simulink model "DF001A_FltInj"  (R2013b)
settings: Solver=FixedStepDiscrete  StartTime=0.0  StopTime=1  FixedStep=.002  RelTol=1e-3
values from neighbouring files (symbols this model uses):
  ARCHGLBPRM_180OVERPI_ULS_F32 = DataDict.Constant    [DF001A_FltInj_DataDict.m]
  ARCHGLBPRM_2PI_ULS_F32 = DataDict.Constant    [DF001A_FltInj_DataDict.m]
  FLOATTOU0P16MULT_ULS_F32 = DataDict.Constant    [DF001A_FltInj_DataDict.m]
  TICNVN_MILLISECPERCNT_F32 = DataDict.Constant    [DF001A_FltInj_DataDict.m]
libraries: simulink x6, NxtrLim x2, NxtrAbslt x1, NxtrMath x1, FixdToFloat x1
(part 1 of 2)
settings Model: PauseTimes=0.198  Creator=qzwc4r  LastModifiedBy=lzz0tm
settings DataIOCC: LimitDataPoints=off  SaveFormat=Structure  ReturnWorkspaceOutputs=on
settings OptimizationCC: BlockReduction=off  InlineParams=on  ZeroExternalMemoryAtStartup=off  ZeroInternalMemoryAtStartup=off  OptimizeModelRefInitCode=on  LifeSpan=1
settings DebuggingCC: SignalInfNanChecking=error  SignalRangeChecking=warning  UnderspecifiedInitializationDetection=Simplified  SolverPrmCheckMsg=error  InheritedTsInSrcMsg=error  DiscreteInheritContinuousMsg=error  SingleTaskRateTransMsg=error  TasksWithSamePriorityMsg=error  SigSpecEnsureSampleTimeMsg=error  CheckMatrixSingularityMsg=error  IntegerOverflowMsg=error  ParameterUnderflowMsg=error  ParameterPrecisionLossMsg=error  ParameterTunabilityLossMsg=error  FixptConstUnderflowMsg=warning  FixptConstOverflowMsg=warning  VectorMatrixConversionMsg=error  SignalLabelMismatchMsg=error  UnconnectedInputMsg=error  UnconnectedOutputMsg=error  UnconnectedLineMsg=error  SFcnCompatibilityMsg=error  UniqueDataStoreMsg=warning  BusObjectLabelMismatch=error  RootOutportRequireBusObject=error  AssertControl=DisableAll  ModelReferenceIOMsg=error  ModelReferenceVersionMismatchMessage=warning  ModelReferenceIOMismatchMessage=error  ModelReferenceCSMismatchMessage=warning  ModelReferenceDataLoggingMessage=error  StateNameClashWarn=warning  StrictBusMsg=ErrorOnBusTreatedAsVector  NonBusSignalsTreatedAsBus=error  SFUnexpectedBacktrackingDiag=error  SFInvalidInputDataAccessInChartInitDiag=error  SFNoUnconditionalDefaultTransitionDiag=error  SFTransitionOutsideNaturalParentDiag=error  SFUnconditionalTransitionShadowingDiag=error  SFUndirectedBroadcastEventsDiag=error
settings ModelReferenceCC: ModelReferenceNumInstancesAllowed=Single
settings RTWCC: SystemTargetFile=autosar.tlc  GenCodeOnly=on  TemplateMakefile=ert_default_tmf  Description=AUTOSAR  GenerateReport=on  ProcessScript=autosar_make_rtw_hook  LaunchReport=on
settings CodeAppCC: GenerateComments=off  IgnoreCustomStorageClasses=off  CustomSymbolStrType=$N$R$M  CustomSymbolStrBlkIO=$N$M  SimulinkBlockComments=off
settings STFCustomTargetCC: ParMdlRefBuildCompliant=on  CompOptLevelCompliant=on  IncludeMdlTerminateFcn=off  CombineOutputUpdateFcns=on  SuppressErrorStatus=on  ERTFirstTimeCompliant=on  ERTCustomFileBanners=on  SupportNonFinite=off  SupportComplex=off  SupportContinuousTime=off  SupportNonInlinedSFcns=off  MATLABClassNameForMDSCustomization=Simulink.SoftwareTarget.ERTCustomization  AutosarCompliant=on  GRTInterface=off  SystemTargetFile=autosar.tlc
settings ERTTargetCC: CodeReplacementLibrary=ANSI_C  ConcurrentExecutionCompliant=off  IncludeMdlTerminateFcn=off  SuppressErrorStatus=on  SupportNonFinite=off  SupportComplex=off  ModelStepFunctionPrototypeControlCompliant=off  CPPClassGenCompliant=off  AutosarCompliant=on  InlinedParameterPlacement=NonHierarchical  ERTCustomFileTemplate=example_file_process.tlc  EnableUserReplacementTypes=on

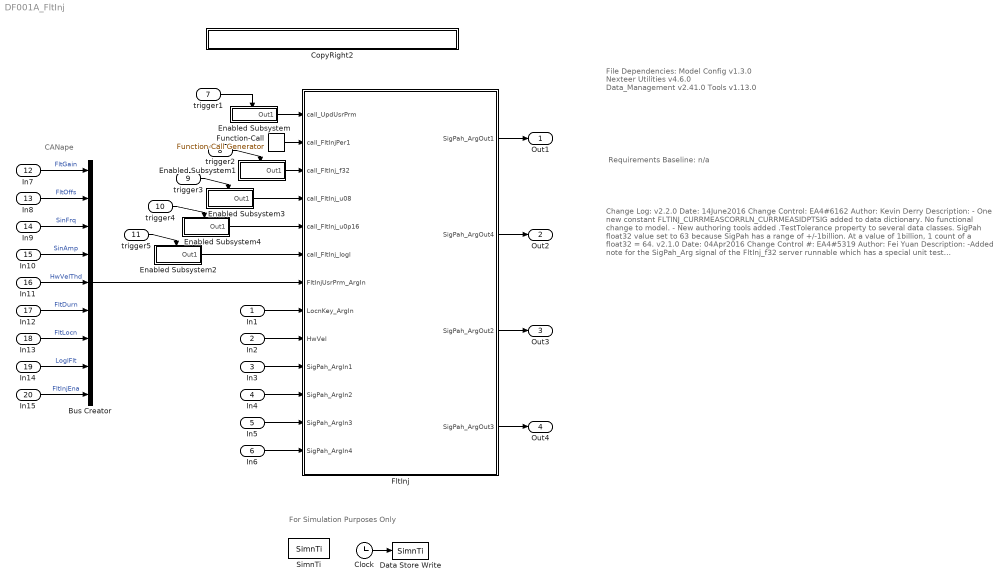
== system DF001A_FltInj ==
  note: CANape
  note: File Dependencies:
      |
      | Model Config v1.3.0
      | Nexteer Utilities v4.6.0
      | Data_Management v2.41.0
      | Tools v1.13.0
  note: Requirements Baseline: n/a
  note: Change Log:
      |
      | v2.2.0
      | Date: 14June2016
      | Change Control:  EA4#6162
      | Author:  Kevin Derry
      | Description:
      | - One new constant FLTINJ_CURRMEASCORRLN_CURRMEASIDPTSIG
      |   added to data dictionary.  No functional change to model.
      | - New authoring tools added .TestTolerance property to several data classes.
      |   SigPah float32 value set to 63 because SigPah has a range of +/-1billion.
      |   At a value of 1billion, 1 count of a float32 = 64.
      |
      | v2.1.0
      | Date: 04Apr2016
      | Change Control #: EA4#5319
      | Author: Fei Yuan
      | Description:
      | -Added note for the SigPah_Arg signal of the FltInj_f32 server runnable
      |  which has a special unit test consideration.
      | - Updated the range for the SigPah_Arg signal of the FltInj_u08 server
      |  runnable to 0-255.
      | - Removed the check for (FltInjUsrPrm.FltInjEna == TRUE) in the
      |   "else if" path.
      | - Added "Cnt" as the DocUnits of FltInjUsrPrm.
      |
      | v2.0.0
      | Change Control #:  EA4#3116
      | Author:  Kevin Derry
      | - New constant FLTINJ_TQOSCN_PREFINALCMD
      | - All constants .DocUnits changed from 'Uls' to 'Cnt' (should
      |   cause no effect on system)
      | - No functional changes to model.
      |
      | v1.1.0
      | Date: 26Aug2015
      | Change Control #: EA4#951
      | Author: Kevin Derry
      | Description:
      | - All InOut server arguments renamed to 'SigPah'.
      | - All PIM names now start with 'FltInj' because code is
      |     really using EA3-style module level variables.
      | - FLOATTOU0P16MULT_ULS_F32 was 65535, now 65536.
      | - Removed all requirements links.
      |
      | v1.0.0
      | Date: 21Aug2015
      | Change Control #: EA4#951
      | Author: Kevin Derry
      | Description:
      | - Initial Release
  note: For Simulation Purposes Only
  In1 : Inport
  In2 : Inport  Port=2
  In3 : Inport  Port=3
  In4 : Inport  Port=4
  In5 : Inport  Port=5
  In6 : Inport  Port=6
  trigger1 : Inport  Port=7
  trigger2 : Inport  Port=8
  trigger3 : Inport  Port=9
  trigger4 : Inport  Port=10
  trigger5 : Inport  Port=11
  In7 : Inport  Port=12
  In8 : Inport  Port=13
  In9 : Inport  Port=14
  In10 : Inport  Port=15
  In11 : Inport  Port=16
  In12 : Inport  Port=17
  In13 : Inport  Port=18
  In14 : Inport  Port=19
  In15 : Inport  Port=20
  Bus Creator : BusCreator  Inputs=9  OutDataTypeStr=Bus: FltInjUsrPrmRec1  NonVirtualBus=on
  Clock : Clock
  CopyRight2 : Subsystem  Description=|  mask(Copyright Information){none=on}
      | Copyright info block.                                               
      |                                                                     
      | Place copyright information at the top of every subsystem in design.
      mask prompts: none "No parameters"
      mask help: Place copyright information at the top of every subsystem in design.
      mask Display:
      | NxtrConf = 'Nexteer Confidential';
      | 
      | sys = bdroot; %handle for the current model ("system")
      | first = get_param(sys,'Created');
      | if(isempty(first))
      |     first = datestr(now,'yyyy');
      | else
      |     first = first(end-3:end);  %year is last four digits
      | end
      | 
      | last = get_param(sys,'LastModifiedDate');
      | if isempty(last)
      |     last = datestr(now,'yyyy');
      | else
      |     last = last(end-3:end);
      | end
      | 
      | if strcmp(first,last)
      |     fprintf('%s -- Copyright %s Nexteer',NxtrConf,first)
      | else
      |     fprintf('%s -- %s%s- %s Nexteer',NxtrConf,char(169),first,last)
      | end
  Data Store Write : DataStoreWrite  DataStoreName=SimnTi
  Enabled Subsystem : Subsystem  TreatAsAtomicUnit=on
  Enabled Subsystem1 : Subsystem  TreatAsAtomicUnit=on
  Enabled Subsystem2 : Subsystem  TreatAsAtomicUnit=on
  Enabled Subsystem3 : Subsystem  TreatAsAtomicUnit=on
  Enabled Subsystem4 : Subsystem  TreatAsAtomicUnit=on
  FltInj : Subsystem
      settings: AttributesFormatString=%<Tag>
  Function-Call : simulink/Ports & Subsystems/Function-Call Generator  sample_time=.002  numberOfIterations=1
  SimnTi : DataStoreMemory  DataStoreName=SimnTi
  Out1 : Outport
  Out2 : Outport  Port=2
  Out3 : Outport  Port=3
  Out4 : Outport  Port=4
  wires:
  Bus Creator/1 -> FltInj/7(FltInjUsrPrm_ArgIn)
  FltInj/1(SigPah_ArgOut1) -> Out1/1
  FltInj/2(SigPah_ArgOut4) -> Out2/1
  Function-Call/1 -> FltInj/2(call_FltInjPer1)
  Enabled Subsystem/1(Out1) -> FltInj/1(call_UpdUsrPrm)
  Enabled Subsystem1/1(Out1) -> FltInj/3(call_FltInj_f32)
  Enabled Subsystem2/1(Out1) -> FltInj/6(call_FltInj_logl)
  In3/1 -> FltInj/10(SigPah_ArgIn1)
  In1/1 -> FltInj/8(LocnKey_ArgIn)
  In2/1 -> FltInj/9(HwVel)
  In6/1 -> FltInj/13(SigPah_ArgIn4)
  Clock/1 -> Data Store Write/1
  FltInj/3(SigPah_ArgOut2) -> Out3/1
  FltInj/4(SigPah_ArgOut3) -> Out4/1
  Enabled Subsystem3/1(Out1) -> FltInj/4(call_FltInj_u08)
  Enabled Subsystem4/1(Out1) -> FltInj/5(call_FltInj_u0p16)
  trigger1/1 -> Enabled Subsystem/Enable
  trigger2/1 -> Enabled Subsystem1/Enable
  trigger3/1 -> Enabled Subsystem3/Enable
  trigger4/1 -> Enabled Subsystem4/Enable
  trigger5/1 -> Enabled Subsystem2/Enable
  In4/1 -> FltInj/11(SigPah_ArgIn2)
  In5/1 -> FltInj/12(SigPah_ArgIn3)
  In15/1 -> Bus Creator/9  "FltInjEna"
  In14/1 -> Bus Creator/8  "LoglFlt"
  In10/1 -> Bus Creator/4  "SinAmp"
  In9/1 -> Bus Creator/3  "SinFrq"
  In8/1 -> Bus Creator/2  "FltOffs"
  In7/1 -> Bus Creator/1  "FltGain"
  In11/1 -> Bus Creator/5  "HwVelThd"
  In12/1 -> Bus Creator/6  "FltDurn"
  In13/1 -> Bus Creator/7  "FltLocn"

== system DF001A_FltInj/CopyRight2 ==

== system DF001A_FltInj/Enabled Subsystem ==
  Enable : EnablePort
  Function-Call : simulink/Ports & Subsystems/Function-Call Generator  sample_time=.002  numberOfIterations=1
  Out1 : Outport
  wires:
  Function-Call/1 -> Out1/1

== system DF001A_FltInj/Enabled Subsystem1 ==
  Enable : EnablePort
  Function-Call : simulink/Ports & Subsystems/Function-Call Generator  sample_time=.002  numberOfIterations=1
  Out1 : Outport
  wires:
  Function-Call/1 -> Out1/1

== system DF001A_FltInj/Enabled Subsystem2 ==
  Enable : EnablePort
  Function-Call : simulink/Ports & Subsystems/Function-Call Generator  sample_time=.002  numberOfIterations=1
  Out1 : Outport
  wires:
  Function-Call/1 -> Out1/1

== system DF001A_FltInj/Enabled Subsystem3 ==
  Enable : EnablePort
  Function-Call : simulink/Ports & Subsystems/Function-Call Generator  sample_time=.002  numberOfIterations=1
  Out1 : Outport
  wires:
  Function-Call/1 -> Out1/1

== system DF001A_FltInj/Enabled Subsystem4 ==
  Enable : EnablePort
  Function-Call : simulink/Ports & Subsystems/Function-Call Generator  sample_time=.002  numberOfIterations=1
  Out1 : Outport
  wires:
  Function-Call/1 -> Out1/1

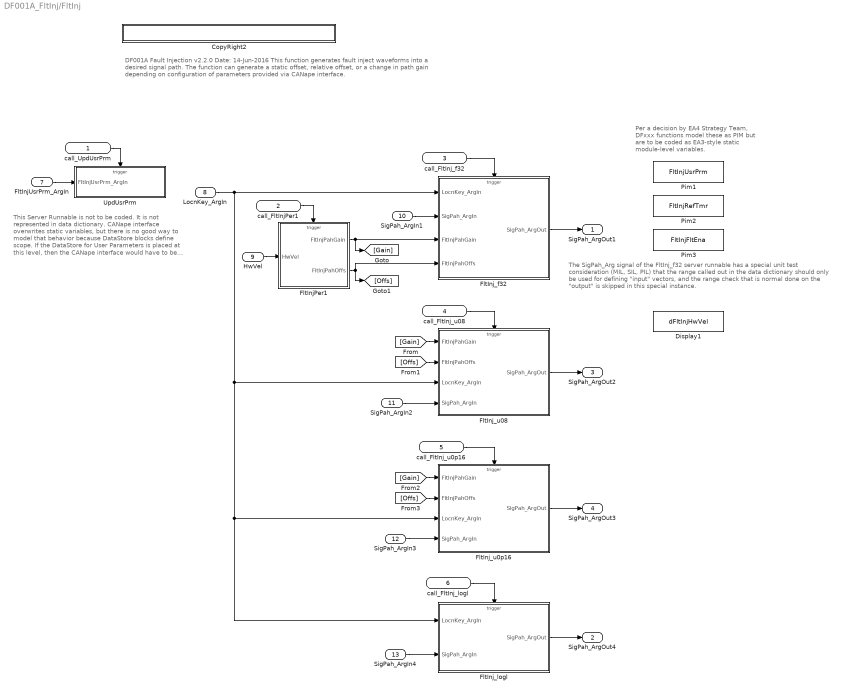
== system DF001A_FltInj/FltInj ==
  note: The SigPah_Arg signal of the FltInj_f32 server runnable has a special unit test
      | consideration (MIL, SIL, PIL) that the range called out in the data dictionary
      | should only be used for defining "input" vectors, and the range check that is normal
      |  done on the "output" is skipped in this special instance.
  note: Per a decision by EA4 Strategy Team,
      | DFxxx functions model these as PIM
      | but are to be coded as EA3-style
      | static module-level variables.
  note: This Server Runnable is not to be coded.
      | It is not represented in data dictionary.
      | CANape interface overwrites static variables,
      | but there is no good way to model that behavior
      | because DataStore blocks define scope.  If the
      | DataStore for User Parameters is placed at this
      | level, then the CANape interface would have to
      | be modeled at this level (inside the component).
  note: DF001A  Fault Injection
      | v2.2.0      Date: 14-Jun-2016
      |
      | This function generates fault inject waveforms into a desired signal path.  The function can generate a static offset, relative offset,
      | or a change in path gain depending on configuration of parameters provided via CANape interface.
  call_UpdUsrPrm : Inport
  call_FltInjPer1 : Inport  RequirementInfo={} %GIDa_20e234b7_6337_4616_ac07_9d9d8320cb43  Port=2
  call_FltInj_f32 : Inport  Port=3
  call_FltInj_u08 : Inport  Port=4
  call_FltInj_u0p16 : Inport  Port=5
  call_FltInj_logl : Inport  Port=6
  FltInjUsrPrm_ArgIn : Inport  Port=7
  LocnKey_ArgIn : Inport  Port=8
  HwVel : Inport  Port=9
  SigPah_ArgIn1 : Inport  Port=10
  SigPah_ArgIn2 : Inport  Port=11
  SigPah_ArgIn3 : Inport  Port=12
  SigPah_ArgIn4 : Inport  Port=13
  CopyRight2 : Subsystem  Description=|  mask(Copyright Information){none=on}
      | Copyright info block.                                               
      |                                                                     
      | Place copyright information at the top of every subsystem in design.
      mask prompts: none "No parameters"
      mask help: Place copyright information at the top of every subsystem in design.
      mask Display:
      | NxtrConf = 'Nexteer Confidential';
      | 
      | sys = bdroot; %handle for the current model ("system")
      | first = get_param(sys,'Created');
      | if(isempty(first))
      |     first = datestr(now,'yyyy');
      | else
      |     first = first(end-3:end);  %year is last four digits
      | end
      | 
      | last = get_param(sys,'LastModifiedDate');
      | if isempty(last)
      |     last = datestr(now,'yyyy');
      | else
      |     last = last(end-3:end);
      | end
      | 
      | if strcmp(first,last)
      |     fprintf('%s -- Copyright %s Nexteer',NxtrConf,first)
      | else
      |     fprintf('%s -- %s%s- %s Nexteer',NxtrConf,char(169),first,last)
      | end
  Display1 : DataStoreMemory  DataStoreName=dFltInjHwVel  StateMustResolveToSignalObject=on
  FltInjPer1 : Subsystem  TreatAsAtomicUnit=on
  FltInj_f32 : Subsystem  RequirementInfo={} %GIDa_5c1ea264_a025_437d_95d1_f9710e716a9a  TreatAsAtomicUnit=on
  FltInj_logl : Subsystem  RequirementInfo={} %GIDa_561801b9_9dd3_498d_bd68_f9a4e32fc01f  TreatAsAtomicUnit=on
  FltInj_u08 : Subsystem  RequirementInfo={} %GIDa_ed5ddef9_be48_44cf_93bb_1e098111485b  TreatAsAtomicUnit=on
  FltInj_u0p16 : Subsystem  RequirementInfo={} %GIDa_5fe3668f_00c5_49b6_ae7d_43651472f9f3  TreatAsAtomicUnit=on
  Pim1 : DataStoreMemory  DataStoreName=FltInjUsrPrm  InitialValue=struct('FltGain',single(1),'FltOffs',single(0),'SinFrq',single(0),'SinAmp',single(0),'HwVelThd',single(0),'FltDurn',single(0),'FltLocn',uint16(0),'LoglFlt',false,'FltInjEna',false)  StateMustResolveToSignalObject=on
  Pim2 : DataStoreMemory  DataStoreName=FltInjRefTmr  StateMustResolveToSignalObject=on
  Pim3 : DataStoreMemory  DataStoreName=FltInjFltEna  StateMustResolveToSignalObject=on
  UpdUsrPrm : Subsystem  TreatAsAtomicUnit=on
  SigPah_ArgOut1 : Outport
  SigPah_ArgOut4 : Outport  Port=2
  SigPah_ArgOut2 : Outport  Port=3
  SigPah_ArgOut3 : Outport  Port=4
  wires:
  call_FltInjPer1/1 -> FltInjPer1/Trigger
  call_FltInj_f32/1 -> FltInj_f32/Trigger
  SigPah_ArgIn1/1 -> FltInj_f32/2(SigPah_ArgIn)
  LocnKey_ArgIn/1 -> FltInj_f32/1(LocnKey_ArgIn), FltInj_logl/1(LocnKey_ArgIn), FltInj_u0p16/3(LocnKey_ArgIn), FltInj_u08/3(LocnKey_ArgIn)
  HwVel/1 -> FltInjPer1/1(HwVel)
  FltInjPer1/1(FltInjPahGain) -> FltInj_f32/3(FltInjPahGain), [Gain]
  FltInjPer1/2(FltInjPahOffs) -> FltInj_f32/4(FltInjPahOffs), [Offs]
  call_UpdUsrPrm/1 -> UpdUsrPrm/Trigger
  FltInjUsrPrm_ArgIn/1 -> UpdUsrPrm/1(FltInjUsrPrm_ArgIn)
  call_FltInj_logl/1 -> FltInj_logl/Trigger
  SigPah_ArgIn4/1 -> FltInj_logl/2(SigPah_ArgIn)
  FltInj_f32/1(SigPah_ArgOut) -> SigPah_ArgOut1/1
  FltInj_logl/1(SigPah_ArgOut) -> SigPah_ArgOut4/1
  call_FltInj_u08/1 -> FltInj_u08/Trigger
  SigPah_ArgIn2/1 -> FltInj_u08/4(SigPah_ArgIn)
  FltInj_u08/1(SigPah_ArgOut) -> SigPah_ArgOut2/1
  call_FltInj_u0p16/1 -> FltInj_u0p16/Trigger
  SigPah_ArgIn3/1 -> FltInj_u0p16/4(SigPah_ArgIn)
  FltInj_u0p16/1(SigPah_ArgOut) -> SigPah_ArgOut3/1
  [Gain] -> FltInj_u08/1(FltInjPahGain)
  [Offs] -> FltInj_u08/2(FltInjPahOffs)
  [Gain] -> FltInj_u0p16/1(FltInjPahGain)
  [Offs] -> FltInj_u0p16/2(FltInjPahOffs)

== system DF001A_FltInj/FltInj/CopyRight2 ==

== system DF001A_FltInj/FltInj/FltInjPer1 ==
  note: All functionality of Periodic 1 is contained within preprocessor conditional statement
      | #if ( FLTINJENA == STD_ON )
      |    do stuff
      | else
      |     empty, do-nothing runnable
      | #endif
  HwVel : Inport
  function : TriggerPort  TriggerType=function-call
  CopyRight2 : Subsystem  Description=|  mask(Copyright Information){none=on}
      | Copyright info block.                                               
      |                                                                     
      | Place copyright information at the top of every subsystem in design.
      mask prompts: none "No parameters"
      mask help: Place copyright information at the top of every subsystem in design.
      mask Display:
      | NxtrConf = 'Nexteer Confidential';
      | 
      | sys = bdroot; %handle for the current model ("system")
      | first = get_param(sys,'Created');
      | if(isempty(first))
      |     first = datestr(now,'yyyy');
      | else
      |     first = first(end-3:end);  %year is last four digits
      | end
      | 
      | last = get_param(sys,'LastModifiedDate');
      | if isempty(last)
      |     last = datestr(now,'yyyy');
      | else
      |     last = last(end-3:end);
      | end
      | 
      | if strcmp(first,last)
      |     fprintf('%s -- Copyright %s Nexteer',NxtrConf,first)
      | else
      |     fprintf('%s -- %s%s- %s Nexteer',NxtrConf,char(169),first,last)
      | end
  Per1 Logic : Subsystem  Variant=on
      settings: GeneratePreprocessorConditionals=on
  FltInjPahGain : Outport
  FltInjPahOffs : Outport  Port=2
  wires:
  HwVel/1 -> Per1 Logic/1(HwVel)
  Per1 Logic/1(FltInjPahGain) -> FltInjPahGain/1
  Per1 Logic/2(FltInjPahOffs) -> FltInjPahOffs/1

== system DF001A_FltInj/FltInj/FltInj_f32 ==
  note: All functionality of FltInj_f32 server runnable is contained within preprocessor conditional statement
      | #if ( FLTINJENA == STD_ON )
      |    do stuff
      | else
      |     empty, do-nothing runnable
      | #endif
  LocnKey_ArgIn : Inport  RequirementInfo={} %GIDa_31a623ae_eeb2_4b88_92ee_315eddd3bcf4
  SigPah_ArgIn : Inport  RequirementInfo={} %GIDa_16b024e5_d763_424d_9c5c_ceb40de65f22  Port=2
  FltInjPahGain : Inport  RequirementInfo={} %GIDa_43ebceda_d1cf_4259_b1a5_c70f9fde258c  Port=3
  FltInjPahOffs : Inport  RequirementInfo={} %GIDa_d69a663e_2e99_4704_b030_83a72ce923af  Port=4
  function : TriggerPort  TriggerType=function-call
  " FltInj_f32 Logic" : Subsystem  Variant=on
      settings: GeneratePreprocessorConditionals=on
  CopyRight2 : Subsystem  Description=|  mask(Copyright Information){none=on}
      | Copyright info block.                                               
      |                                                                     
      | Place copyright information at the top of every subsystem in design.
      mask prompts: none "No parameters"
      mask help: Place copyright information at the top of every subsystem in design.
      mask Display:
      | NxtrConf = 'Nexteer Confidential';
      | 
      | sys = bdroot; %handle for the current model ("system")
      | first = get_param(sys,'Created');
      | if(isempty(first))
      |     first = datestr(now,'yyyy');
      | else
      |     first = first(end-3:end);  %year is last four digits
      | end
      | 
      | last = get_param(sys,'LastModifiedDate');
      | if isempty(last)
      |     last = datestr(now,'yyyy');
      | else
      |     last = last(end-3:end);
      | end
      | 
      | if strcmp(first,last)
      |     fprintf('%s -- Copyright %s Nexteer',NxtrConf,first)
      | else
      |     fprintf('%s -- %s%s- %s Nexteer',NxtrConf,char(169),first,last)
      | end
  SigPah_ArgOut : Outport
  wires:
  SigPah_ArgIn/1 -> " FltInj_f32 Logic"/3(SigPah_ArgIn)
  LocnKey_ArgIn/1 -> " FltInj_f32 Logic"/4(LocnKey_ArgIn)
  FltInjPahGain/1 -> " FltInj_f32 Logic"/1(PahGain)
  FltInjPahOffs/1 -> " FltInj_f32 Logic"/2(PahOffs)
  " FltInj_f32 Logic"/1(SigPah_ArgOut) -> SigPah_ArgOut/1

== system DF001A_FltInj/FltInj/FltInj_logl ==
  note: All functionality of FltInj_f32 server runnable is contained within preprocessor conditional statement
      | #if ( FLTINJENA == STD_ON )
      |    do stuff
      | else
      |     empty, do-nothing runnable
      | #endif
  note: FltInj_Lgc
  LocnKey_ArgIn : Inport  RequirementInfo={} %GIDa_2ae7ab17_5d49_468b_b736_51e520c74cd6
  SigPah_ArgIn : Inport  RequirementInfo={} %GIDa_b2acbf61_1294_415e_81b7_5846abe7e02f  Port=2
  function : TriggerPort  TriggerType=function-call
  CopyRight2 : Subsystem  Description=|  mask(Copyright Information){none=on}
      | Copyright info block.                                               
      |                                                                     
      | Place copyright information at the top of every subsystem in design.
      mask prompts: none "No parameters"
      mask help: Place copyright information at the top of every subsystem in design.
      mask Display:
      | NxtrConf = 'Nexteer Confidential';
      | 
      | sys = bdroot; %handle for the current model ("system")
      | first = get_param(sys,'Created');
      | if(isempty(first))
      |     first = datestr(now,'yyyy');
      | else
      |     first = first(end-3:end);  %year is last four digits
      | end
      | 
      | last = get_param(sys,'LastModifiedDate');
      | if isempty(last)
      |     last = datestr(now,'yyyy');
      | else
      |     last = last(end-3:end);
      | end
      | 
      | if strcmp(first,last)
      |     fprintf('%s -- Copyright %s Nexteer',NxtrConf,first)
      | else
      |     fprintf('%s -- %s%s- %s Nexteer',NxtrConf,char(169),first,last)
      | end
  FltInj_lgc Logic : Subsystem  Variant=on
      settings: GeneratePreprocessorConditionals=on
  SigPah_ArgOut : Outport
  wires:
  LocnKey_ArgIn/1 -> FltInj_lgc Logic/1(LocnKey_ArgIn)
  SigPah_ArgIn/1 -> FltInj_lgc Logic/2(SigPah_ArgIn)
  FltInj_lgc Logic/1(SigPah_ArgOut) -> SigPah_ArgOut/1

== system DF001A_FltInj/FltInj/FltInj_u08 ==
  note: All functionality of FltInj_fu08 server runnable is contained within preprocessor conditional statement
      | #if ( FLTINJENA == STD_ON )
      |    do stuff
      | else
      |     empty, do-nothing runnable
      | #endif
  note: FltInj_u08
  note: FltInj_u08
  FltInjPahGain : Inport  RequirementInfo={} %GIDa_c9197515_1ebc_4daa_890f_8bacffcbaee3
  FltInjPahOffs : Inport  RequirementInfo={} %GIDa_0526e46e_f231_4162_99dd_eea93105a2d2  Port=2
  LocnKey_ArgIn : Inport  RequirementInfo={} %GIDa_d188acad_33a8_4158_b174_4092ffeef513  Port=3
  SigPah_ArgIn : Inport  RequirementInfo={} %GIDa_2406ebfe_6cfe_4aa7_b904_2b925d9436a9  Port=4
  function : TriggerPort  TriggerType=function-call
  " FltInj_u08 Logic" : Subsystem  Variant=on
      settings: GeneratePreprocessorConditionals=on
  CopyRight2 : Subsystem  Description=|  mask(Copyright Information){none=on}
      | Copyright info block.                                               
      |                                                                     
      | Place copyright information at the top of every subsystem in design.
      mask prompts: none "No parameters"
      mask help: Place copyright information at the top of every subsystem in design.
      mask Display:
      | NxtrConf = 'Nexteer Confidential';
      | 
      | sys = bdroot; %handle for the current model ("system")
      | first = get_param(sys,'Created');
      | if(isempty(first))
      |     first = datestr(now,'yyyy');
      | else
      |     first = first(end-3:end);  %year is last four digits
      | end
      | 
      | last = get_param(sys,'LastModifiedDate');
      | if isempty(last)
      |     last = datestr(now,'yyyy');
      | else
      |     last = last(end-3:end);
      | end
      | 
      | if strcmp(first,last)
      |     fprintf('%s -- Copyright %s Nexteer',NxtrConf,first)
      | else
      |     fprintf('%s -- %s%s- %s Nexteer',NxtrConf,char(169),first,last)
      | end
  SigPah_ArgOut : Outport
  wires:
  SigPah_ArgIn/1 -> " FltInj_u08 Logic"/3(SigPah_ArgIn)
  LocnKey_ArgIn/1 -> " FltInj_u08 Logic"/4(LocnKey_ArgIn)
  FltInjPahGain/1 -> " FltInj_u08 Logic"/1(PahGain)
  FltInjPahOffs/1 -> " FltInj_u08 Logic"/2(PahOffs)
  " FltInj_u08 Logic"/1(SigPah_ArgOut) -> SigPah_ArgOut/1

== system DF001A_FltInj/FltInj/FltInj_u0p16 ==
  note: All functionality of FltInj_fu08 server runnable is contained within preprocessor conditional statement
      | #if ( FLTINJENA == STD_ON )
      |    do stuff
      | else
      |     empty, do-nothing runnable
      | #endif
  note: FltInj_u0p16
  FltInjPahGain : Inport  RequirementInfo={} %GIDa_eb53d382_c45a_45e2_a75c_eda2fd91d1cd
  FltInjPahOffs : Inport  RequirementInfo={} %GIDa_29c855bb_c0f4_4f29_a054_1b579e9a2ad9  Port=2
  LocnKey_ArgIn : Inport  RequirementInfo={} %GIDa_47dbfc04_082f_4bad_a590_02b3bef71f68  Port=3
  SigPah_ArgIn : Inport  RequirementInfo={} %GIDa_cabac5df_d07f_4daa_8cc9_67b8f83a04f7  Port=4
  function : TriggerPort  TriggerType=function-call
  " FltInj_u0p16 Logic" : Subsystem  Variant=on
      settings: GeneratePreprocessorConditionals=on
  CopyRight2 : Subsystem  Description=|  mask(Copyright Information){none=on}
      | Copyright info block.                                               
      |                                                                     
      | Place copyright information at the top of every subsystem in design.
      mask prompts: none "No parameters"
      mask help: Place copyright information at the top of every subsystem in design.
      mask Display:
      | NxtrConf = 'Nexteer Confidential';
      | 
      | sys = bdroot; %handle for the current model ("system")
      | first = get_param(sys,'Created');
      | if(isempty(first))
      |     first = datestr(now,'yyyy');
      | else
      |     first = first(end-3:end);  %year is last four digits
      | end
      | 
      | last = get_param(sys,'LastModifiedDate');
      | if isempty(last)
      |     last = datestr(now,'yyyy');
      | else
      |     last = last(end-3:end);
      | end
      | 
      | if strcmp(first,last)
      |     fprintf('%s -- Copyright %s Nexteer',NxtrConf,first)
      | else
      |     fprintf('%s -- %s%s- %s Nexteer',NxtrConf,char(169),first,last)
      | end
  SigPah_ArgOut : Outport
  wires:
  SigPah_ArgIn/1 -> " FltInj_u0p16 Logic"/3(SigPah_ArgIn)
  LocnKey_ArgIn/1 -> " FltInj_u0p16 Logic"/4(LocnKey_ArgIn)
  FltInjPahGain/1 -> " FltInj_u0p16 Logic"/1(PahGain)
  FltInjPahOffs/1 -> " FltInj_u0p16 Logic"/2(PahOffs)
  " FltInj_u0p16 Logic"/1(SigPah_ArgOut) -> SigPah_ArgOut/1

== system DF001A_FltInj/FltInj/UpdUsrPrm ==
  FltInjUsrPrm_ArgIn : Inport
  function : TriggerPort  TriggerType=function-call
  CopyRight2 : Subsystem  Description=|  mask(Copyright Information){none=on}
      | Copyright info block.                                               
      |                                                                     
      | Place copyright information at the top of every subsystem in design.
      mask prompts: none "No parameters"
      mask help: Place copyright information at the top of every subsystem in design.
      mask Display:
      | NxtrConf = 'Nexteer Confidential';
      | 
      | sys = bdroot; %handle for the current model ("system")
      | first = get_param(sys,'Created');
      | if(isempty(first))
      |     first = datestr(now,'yyyy');
      | else
      |     first = first(end-3:end);  %year is last four digits
      | end
      | 
      | last = get_param(sys,'LastModifiedDate');
      | if isempty(last)
      |     last = datestr(now,'yyyy');
      | else
      |     last = last(end-3:end);
      | end
      | 
      | if strcmp(first,last)
      |     fprintf('%s -- Copyright %s Nexteer',NxtrConf,first)
      | else
      |     fprintf('%s -- %s%s- %s Nexteer',NxtrConf,char(169),first,last)
      | end
  Data Store Write : DataStoreWrite  DataStoreName=FltInjUsrPrm
  wires:
  FltInjUsrPrm_ArgIn/1 -> Data Store Write/1

== system DF001A_FltInj/FltInj/FltInjPer1/CopyRight2 ==

== system DF001A_FltInj/FltInj/FltInjPer1/Per1 Logic ==
  note: 1) Only subsystems can be added as variant choices at this level
      | 2) Blocks cannot be connected at this level as connectivity is
      | automatically determined at simulation, based on the active variant
  HwVel : Inport
  CopyRight2 : Subsystem  Description=|  mask(Copyright Information){none=on}
      | Copyright info block.                                               
      |                                                                     
      | Place copyright information at the top of every subsystem in design.
      mask prompts: none "No parameters"
      mask help: Place copyright information at the top of every subsystem in design.
      mask Display:
      | NxtrConf = 'Nexteer Confidential';
      | 
      | sys = bdroot; %handle for the current model ("system")
      | first = get_param(sys,'Created');
      | if(isempty(first))
      |     first = datestr(now,'yyyy');
      | else
      |     first = first(end-3:end);  %year is last four digits
      | end
      | 
      | last = get_param(sys,'LastModifiedDate');
      | if isempty(last)
      |     last = datestr(now,'yyyy');
      | else
      |     last = last(end-3:end);
      | end
      | 
      | if strcmp(first,last)
      |     fprintf('%s -- Copyright %s Nexteer',NxtrConf,first)
      | else
      |     fprintf('%s -- %s%s- %s Nexteer',NxtrConf,char(169),first,last)
      | end
  ProductionBuild : Subsystem  VariantControl=FLTINJENA ~= STD_ON
  SpecialBuild : Subsystem  VariantControl=FLTINJENA == STD_ON
  FltInjPahGain : Outport
  FltInjPahOffs : Outport  Port=2

== system DF001A_FltInj/FltInj/FltInj_f32/ FltInj_f32 Logic ==
  note: 1) Only subsystems can be added as variant choices at this level
      | 2) Blocks cannot be connected at this level as connectivity is
      | automatically determined at simulation, based on the active variant
  PahGain : Inport  RequirementInfo={} %GIDa_5636614f_0456_4eb8_a790_b6c0e06a38e3
  PahOffs : Inport  RequirementInfo={} %GIDa_4aacf5bc_4ebb_470e_be11_f3ae4130ab3a  Port=2
  SigPah_ArgIn : Inport  RequirementInfo={} %GIDa_ed33cccd_a3a6_443e_9d97_9ecff4ba9cf2  Port=3
  LocnKey_ArgIn : Inport  RequirementInfo={} %GIDa_37d705d6_a2de_43e2_9706_d808a393d6c2  Port=4
  CopyRight2 : Subsystem  Description=|  mask(Copyright Information){none=on}
      | Copyright info block.                                               
      |                                                                     
      | Place copyright information at the top of every subsystem in design.
      mask prompts: none "No parameters"
      mask help: Place copyright information at the top of every subsystem in design.
      mask Display:
      | NxtrConf = 'Nexteer Confidential';
      | 
      | sys = bdroot; %handle for the current model ("system")
      | first = get_param(sys,'Created');
      | if(isempty(first))
      |     first = datestr(now,'yyyy');
      | else
      |     first = first(end-3:end);  %year is last four digits
      | end
      | 
      | last = get_param(sys,'LastModifiedDate');
      | if isempty(last)
      |     last = datestr(now,'yyyy');
      | else
      |     last = last(end-3:end);
      | end
      | 
      | if strcmp(first,last)
      |     fprintf('%s -- Copyright %s Nexteer',NxtrConf,first)
      | else
      |     fprintf('%s -- %s%s- %s Nexteer',NxtrConf,char(169),first,last)
      | end
  ProductionBuild : Subsystem  VariantControl=FLTINJENA ~= STD_ON
  SpecialBuild : Subsystem  VariantControl=FLTINJENA == STD_ON
  SigPah_ArgOut : Outport

== system DF001A_FltInj/FltInj/FltInj_f32/CopyRight2 ==

== system DF001A_FltInj/FltInj/FltInj_logl/CopyRight2 ==

== system DF001A_FltInj/FltInj/FltInj_logl/FltInj_lgc Logic ==
  note: 1) Only subsystems can be added as variant choices at this level
      | 2) Blocks cannot be connected at this level as connectivity is
      | automatically determined at simulation, based on the active variant
  note: FltInj_Lgc
  LocnKey_ArgIn : Inport  RequirementInfo={} %GIDa_55c95650_e774_4272_814a_52a3b2f4bd8f
  SigPah_ArgIn : Inport  RequirementInfo={} %GIDa_9314202e_4dc8_4baf_92ae_0d4e8fbb5b3c  Port=2
  CopyRight2 : Subsystem  Description=|  mask(Copyright Information){none=on}
      | Copyright info block.                                               
      |                                                                     
      | Place copyright information at the top of every subsystem in design.
      mask prompts: none "No parameters"
      mask help: Place copyright information at the top of every subsystem in design.
      mask Display:
      | NxtrConf = 'Nexteer Confidential';
      | 
      | sys = bdroot; %handle for the current model ("system")
      | first = get_param(sys,'Created');
      | if(isempty(first))
      |     first = datestr(now,'yyyy');
      | else
      |     first = first(end-3:end);  %year is last four digits
      | end
      | 
      | last = get_param(sys,'LastModifiedDate');
      | if isempty(last)
      |     last = datestr(now,'yyyy');
      | else
      |     last = last(end-3:end);
      | end
      | 
      | if strcmp(first,last)
      |     fprintf('%s -- Copyright %s Nexteer',NxtrConf,first)
      | else
      |     fprintf('%s -- %s%s- %s Nexteer',NxtrConf,char(169),first,last)
      | end
  ProductionBuild : Subsystem  VariantControl=FLTINJENA ~= STD_ON
  SpecialBuild : Subsystem  VariantControl=FLTINJENA == STD_ON
  SigPah_ArgOut : Outport

== system DF001A_FltInj/FltInj/FltInj_u08/ FltInj_u08 Logic ==
  note: 1) Only subsystems can be added as variant choices at this level
      | 2) Blocks cannot be connected at this level as connectivity is
      | automatically determined at simulation, based on the active variant
  note: FltInj_u08
  PahGain : Inport  RequirementInfo={} %GIDa_075396eb_862a_4290_8684_2489e579a359
  PahOffs : Inport  RequirementInfo={} %GIDa_6c474b44_151c_4e58_845f_c03e430ca976  Port=2
  SigPah_ArgIn : Inport  RequirementInfo={} %GIDa_ef123915_cf98_46ee_976a_5eec4739c2d7  Port=3
  LocnKey_ArgIn : Inport  RequirementInfo={} %GIDa_ddb5076c_817d_4e1f_a555_42f98f3cee51  Port=4
  CopyRight2 : Subsystem  Description=|  mask(Copyright Information){none=on}
      | Copyright info block.                                               
      |                                                                     
      | Place copyright information at the top of every subsystem in design.
      mask prompts: none "No parameters"
      mask help: Place copyright information at the top of every subsystem in design.
      mask Display:
      | NxtrConf = 'Nexteer Confidential';
      | 
      | sys = bdroot; %handle for the current model ("system")
      | first = get_param(sys,'Created');
      | if(isempty(first))
      |     first = datestr(now,'yyyy');
      | else
      |     first = first(end-3:end);  %year is last four digits
      | end
      | 
      | last = get_param(sys,'LastModifiedDate');
      | if isempty(last)
      |     last = datestr(now,'yyyy');
      | else
      |     last = last(end-3:end);
      | end
      | 
      | if strcmp(first,last)
      |     fprintf('%s -- Copyright %s Nexteer',NxtrConf,first)
      | else
      |     fprintf('%s -- %s%s- %s Nexteer',NxtrConf,char(169),first,last)
      | end
  ProductionBuild : Subsystem  VariantControl=FLTINJENA ~= STD_ON
  SpecialBuild : Subsystem  VariantControl=FLTINJENA == STD_ON
  SigPah_ArgOut : Outport

== system DF001A_FltInj/FltInj/FltInj_u08/CopyRight2 ==

== system DF001A_FltInj/FltInj/FltInj_u0p16/ FltInj_u0p16 Logic ==
  note: 1) Only subsystems can be added as variant choices at this level
      | 2) Blocks cannot be connected at this level as connectivity is
      | automatically determined at simulation, based on the active variant
  note: FltInj_u0p16
  PahGain : Inport  RequirementInfo={} %GIDa_37e8d4cf_a147_408a_982e_1c56467170f5
  PahOffs : Inport  RequirementInfo={} %GIDa_3f375aa8_bf67_457b_8dcd_462917b6a261  Port=2
  SigPah_ArgIn : Inport  RequirementInfo={} %GIDa_5ac97fda_be50_42ae_b664_0a547c6bf129  Port=3
  LocnKey_ArgIn : Inport  RequirementInfo={} %GIDa_d96406ba_8074_4d20_8ab1_a362fc0ebbb7  Port=4
  CopyRight2 : Subsystem  Description=|  mask(Copyright Information){none=on}
      | Copyright info block.                                               
      |                                                                     
      | Place copyright information at the top of every subsystem in design.
      mask prompts: none "No parameters"
      mask help: Place copyright information at the top of every subsystem in design.
      mask Display:
      | NxtrConf = 'Nexteer Confidential';
      | 
      | sys = bdroot; %handle for the current model ("system")
      | first = get_param(sys,'Created');
      | if(isempty(first))
      |     first = datestr(now,'yyyy');
      | else
      |     first = first(end-3:end);  %year is last four digits
      | end
      | 
      | last = get_param(sys,'LastModifiedDate');
      | if isempty(last)
      |     last = datestr(now,'yyyy');
      | else
      |     last = last(end-3:end);
      | end
      | 
      | if strcmp(first,last)
      |     fprintf('%s -- Copyright %s Nexteer',NxtrConf,first)
      | else
      |     fprintf('%s -- %s%s- %s Nexteer',NxtrConf,char(169),first,last)
      | end
  ProductionBuild : Subsystem  VariantControl=FLTINJENA ~= STD_ON
  SpecialBuild : Subsystem  VariantControl=FLTINJENA == STD_ON
  SigPah_ArgOut : Outport

== system DF001A_FltInj/FltInj/FltInj_u0p16/CopyRight2 ==

== system DF001A_FltInj/FltInj/UpdUsrPrm/CopyRight2 ==

== system DF001A_FltInj/FltInj/FltInjPer1/Per1 Logic/CopyRight2 ==

== system DF001A_FltInj/FltInj/FltInjPer1/Per1 Logic/ProductionBuild ==
  HwVel : Inport
  CopyRight2 : Subsystem  Description=|  mask(Copyright Information){none=on}
      | Copyright info block.                                               
      |                                                                     
      | Place copyright information at the top of every subsystem in design.
      mask prompts: none "No parameters"
      mask help: Place copyright information at the top of every subsystem in design.
      mask Display:
      | NxtrConf = 'Nexteer Confidential';
      | 
      | sys = bdroot; %handle for the current model ("system")
      | first = get_param(sys,'Created');
      | if(isempty(first))
      |     first = datestr(now,'yyyy');
      | else
      |     first = first(end-3:end);  %year is last four digits
      | end
      | 
      | last = get_param(sys,'LastModifiedDate');
      | if isempty(last)
      |     last = datestr(now,'yyyy');
      | else
      |     last = last(end-3:end);
      | end
      | 
      | if strcmp(first,last)
      |     fprintf('%s -- Copyright %s Nexteer',NxtrConf,first)
      | else
      |     fprintf('%s -- %s%s- %s Nexteer',NxtrConf,char(169),first,last)
      | end
  Ground1 : Ground
  Ground2 : Ground
  Terminator : Terminator
  FltInjPahGain : Outport
  FltInjPahOffs : Outport  Port=2
  wires:
  HwVel/1 -> Terminator/1
  Ground1/1 -> FltInjPahGain/1
  Ground2/1 -> FltInjPahOffs/1

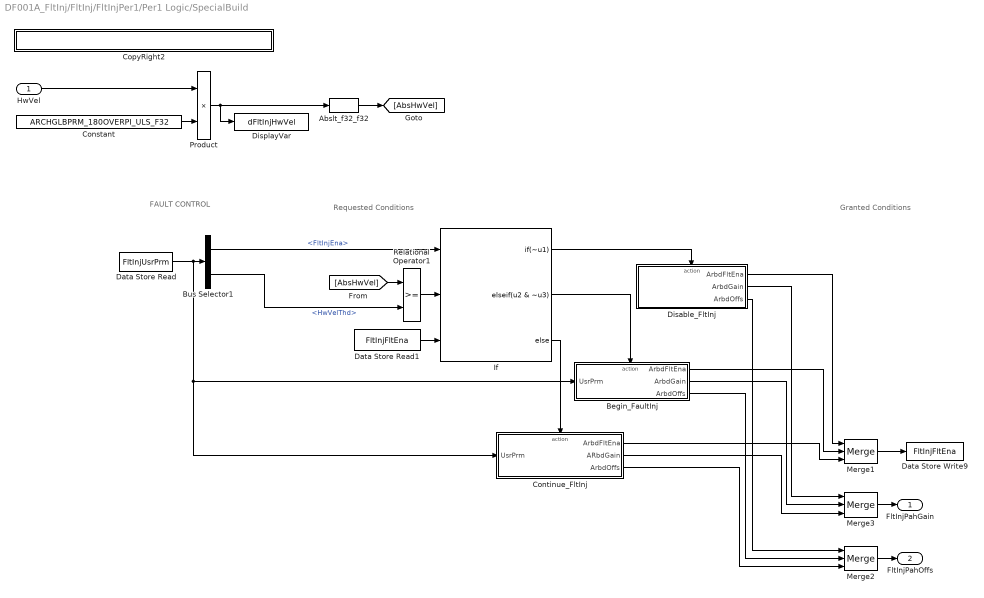
== system DF001A_FltInj/FltInj/FltInjPer1/Per1 Logic/SpecialBuild ==
  note: Requested Conditions
  note: FAULT CONTROL
  note: Granted Conditions
  HwVel : Inport
  Abslt_f32_f32 : NxtrAbslt/Abslt_f32_f32  SFunctionSpec=single y1 = Abslt_f32_f32(single u1)
      settings: AttributesFormatString=%<Name>
  Begin_FaultInj : Subsystem  TreatAsAtomicUnit=on
  Bus Selector1 : BusSelector  OutputSignals=FltInjEna,HwVelThd
  Constant : Constant  Value=ARCHGLBPRM_180OVERPI_ULS_F32
  Continue_FltInj : Subsystem  TreatAsAtomicUnit=on
  CopyRight2 : Subsystem  Description=|  mask(Copyright Information){none=on}
      | Copyright info block.                                               
      |                                                                     
      | Place copyright information at the top of every subsystem in design.
      mask prompts: none "No parameters"
      mask help: Place copyright information at the top of every subsystem in design.
      mask Display:
      | NxtrConf = 'Nexteer Confidential';
      | 
      | sys = bdroot; %handle for the current model ("system")
      | first = get_param(sys,'Created');
      | if(isempty(first))
      |     first = datestr(now,'yyyy');
      | else
      |     first = first(end-3:end);  %year is last four digits
      | end
      | 
      | last = get_param(sys,'LastModifiedDate');
      | if isempty(last)
      |     last = datestr(now,'yyyy');
      | else
      |     last = last(end-3:end);
      | end
      | 
      | if strcmp(first,last)
      |     fprintf('%s -- Copyright %s Nexteer',NxtrConf,first)
      | else
      |     fprintf('%s -- %s%s- %s Nexteer',NxtrConf,char(169),first,last)
      | end
  Data Store Read : DataStoreRead  DataStoreName=FltInjUsrPrm
  Data Store Read1 : DataStoreRead  DataStoreName=FltInjFltEna
  Data Store Write9 : DataStoreWrite  DataStoreName=FltInjFltEna
  Disable_FltInj : Subsystem  TreatAsAtomicUnit=on
  DisplayVar : DataStoreWrite  DataStoreName=dFltInjHwVel
  If : If  NumInputs=3  IfExpression=~u1  ElseIfExpressions=u2 & ~u3
  Merge1 : Merge  Inputs=3
  Merge2 : Merge  Inputs=3
  Merge3 : Merge  Inputs=3
  Product : Product
  Relational Operator1 : RelationalOperator  OutDataTypeStr=boolean
  FltInjPahGain : Outport
  FltInjPahOffs : Outport  Port=2
  wires:
  Data Store Read1/1 -> If/3
  Bus Selector1/1 -> If/1  "<FltInjEna>"
  Bus Selector1/2 -> Relational Operator1/2  "<HwVelThd>"
  [AbsHwVel] -> Relational Operator1/1
  Relational Operator1/1 -> If/2
  If/1 -> Disable_FltInj/Action
  If/2 -> Begin_FaultInj/Action
  If/3 -> Continue_FltInj/Action
  Merge1/1 -> Data Store Write9/1
  Merge3/1 -> FltInjPahGain/1
  Data Store Read/1 -> Continue_FltInj/1(UsrPrm), Begin_FaultInj/1(UsrPrm), Bus Selector1/1
  Disable_FltInj/1(ArbdFltEna) -> Merge1/1
  Begin_FaultInj/1(ArbdFltEna) -> Merge1/2
  Continue_FltInj/1(ArbdFltEna) -> Merge1/3
  Begin_FaultInj/2(ArbdGain) -> Merge3/2
  Disable_FltInj/2(ArbdGain) -> Merge3/1
  Continue_FltInj/2(ARbdGain) -> Merge3/3
  Continue_FltInj/3(ArbdOffs) -> Merge2/3
  Begin_FaultInj/3(ArbdOffs) -> Merge2/2
  Disable_FltInj/3(ArbdOffs) -> Merge2/1
  Merge2/1 -> FltInjPahOffs/1
  HwVel/1 -> Product/1
  Constant/1 -> Product/2
  Product/1 -> DisplayVar/1, Abslt_f32_f32/1
  Abslt_f32_f32/1 -> [AbsHwVel]

== system DF001A_FltInj/FltInj/FltInj_f32/ FltInj_f32 Logic/CopyRight2 ==

== system DF001A_FltInj/FltInj/FltInj_f32/ FltInj_f32 Logic/ProductionBuild ==
  PahGain : Inport  RequirementInfo={} %GIDa_ed8b5d4a_6a58_494c_892f_35987a498b9a
  PahOffs : Inport  RequirementInfo={} %GIDa_d1afa286_5cc7_4336_a084_ae978ab71751  Port=2
  SigPah_ArgIn : Inport  RequirementInfo={} %GIDa_68ab1126_6b55_40bd_b28f_7133ad07e604  Port=3
  LocnKey_ArgIn : Inport  RequirementInfo={} %GIDa_4dbe7e86_cf60_408b_af3d_4633fd32aac1  Port=4
  CopyRight2 : Subsystem  Description=|  mask(Copyright Information){none=on}
      | Copyright info block.                                               
      |                                                                     
      | Place copyright information at the top of every subsystem in design.
      mask prompts: none "No parameters"
      mask help: Place copyright information at the top of every subsystem in design.
      mask Display:
      | NxtrConf = 'Nexteer Confidential';
      | 
      | sys = bdroot; %handle for the current model ("system")
      | first = get_param(sys,'Created');
      | if(isempty(first))
      |     first = datestr(now,'yyyy');
      | else
      |     first = first(end-3:end);  %year is last four digits
      | end
      | 
      | last = get_param(sys,'LastModifiedDate');
      | if isempty(last)
      |     last = datestr(now,'yyyy');
      | else
      |     last = last(end-3:end);
      | end
      | 
      | if strcmp(first,last)
      |     fprintf('%s -- Copyright %s Nexteer',NxtrConf,first)
      | else
      |     fprintf('%s -- %s%s- %s Nexteer',NxtrConf,char(169),first,last)
      | end
  Ground : Ground
  Terminator{,1,3..4} (4 alike) : Terminator
  SigPah_ArgOut : Outport
  wires:
  PahGain/1 -> Terminator/1
  PahOffs/1 -> Terminator1/1
  SigPah_ArgIn/1 -> Terminator3/1
  LocnKey_ArgIn/1 -> Terminator4/1
  Ground/1 -> SigPah_ArgOut/1

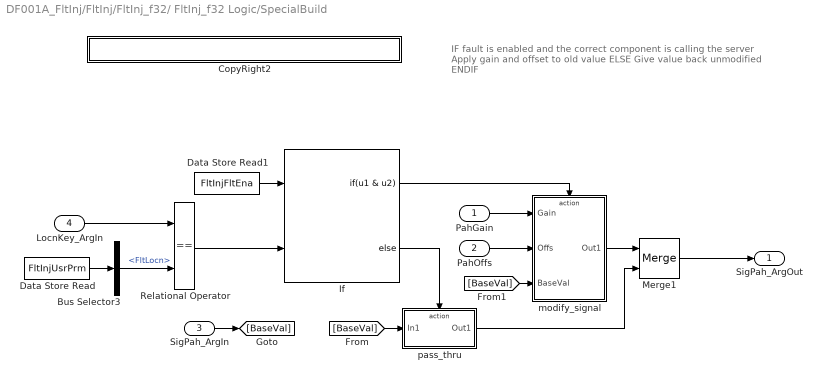
== system DF001A_FltInj/FltInj/FltInj_f32/ FltInj_f32 Logic/SpecialBuild ==
  note: IF  fault is enabled and the correct component is calling the server
      |     Apply gain and offset to old value
      | ELSE
      |     Give value back unmodified
      | ENDIF
  PahGain : Inport  RequirementInfo={} %GIDa_72cfae2d_851b_4294_9b3a_620c4ceeccbe
  PahOffs : Inport  RequirementInfo={} %GIDa_0e8c86da_0b85_49cc_9564_c6f91311e6d3  Port=2
  SigPah_ArgIn : Inport  RequirementInfo={} %GIDa_e3640573_7592_4f4a_93d3_0feb5a441ab4  Port=3
  LocnKey_ArgIn : Inport  RequirementInfo={} %GIDa_511f7dc9_5cae_4553_a845_e3af894b3ec3  Port=4
  Bus Selector3 : BusSelector  OutputSignals=FltLocn
  CopyRight2 : Subsystem  Description=|  mask(Copyright Information){none=on}
      | Copyright info block.                                               
      |                                                                     
      | Place copyright information at the top of every subsystem in design.
      mask prompts: none "No parameters"
      mask help: Place copyright information at the top of every subsystem in design.
      mask Display:
      | NxtrConf = 'Nexteer Confidential';
      | 
      | sys = bdroot; %handle for the current model ("system")
      | first = get_param(sys,'Created');
      | if(isempty(first))
      |     first = datestr(now,'yyyy');
      | else
      |     first = first(end-3:end);  %year is last four digits
      | end
      | 
      | last = get_param(sys,'LastModifiedDate');
      | if isempty(last)
      |     last = datestr(now,'yyyy');
      | else
      |     last = last(end-3:end);
      | end
      | 
      | if strcmp(first,last)
      |     fprintf('%s -- Copyright %s Nexteer',NxtrConf,first)
      | else
      |     fprintf('%s -- %s%s- %s Nexteer',NxtrConf,char(169),first,last)
      | end
  Data Store Read : DataStoreRead  DataStoreName=FltInjUsrPrm
  Data Store Read1 : DataStoreRead  DataStoreName=FltInjFltEna
  If : If  NumInputs=2  IfExpression=u1 & u2
  Merge1 : Merge
  Relational Operator : RelationalOperator  Operator===
  modify_signal : Subsystem  TreatAsAtomicUnit=on
  pass_thru : Subsystem  TreatAsAtomicUnit=on
  SigPah_ArgOut : Outport
  wires:
  Merge1/1 -> SigPah_ArgOut/1
  Data Store Read/1 -> Bus Selector3/1
  PahGain/1 -> modify_signal/1(Gain)
  PahOffs/1 -> modify_signal/2(Offs)
  SigPah_ArgIn/1 -> [BaseVal]
  [BaseVal] -> pass_thru/1(In1)
  [BaseVal] -> modify_signal/3(BaseVal)
  If/1 -> modify_signal/Action
  If/2 -> pass_thru/Action
  modify_signal/1(Out1) -> Merge1/1
  pass_thru/1(Out1) -> Merge1/2
  Data Store Read1/1 -> If/1
  LocnKey_ArgIn/1 -> Relational Operator/1
  Bus Selector3/1 -> Relational Operator/2  "<FltLocn>"
  Relational Operator/1 -> If/2

== system DF001A_FltInj/FltInj/FltInj_logl/FltInj_lgc Logic/CopyRight2 ==

== system DF001A_FltInj/FltInj/FltInj_logl/FltInj_lgc Logic/ProductionBuild ==
  LocnKey_ArgIn : Inport  RequirementInfo={} %GIDa_b5ee89c0_4420_439b_a4ea_75e34a9a42b5
  SigPah_ArgIn : Inport  RequirementInfo={} %GIDa_c6f57e85_979b_48c1_9e55_03af27f58960  Port=2
  CopyRight2 : Subsystem  Description=|  mask(Copyright Information){none=on}
      | Copyright info block.                                               
      |                                                                     
      | Place copyright information at the top of every subsystem in design.
      mask prompts: none "No parameters"
      mask help: Place copyright information at the top of every subsystem in design.
      mask Display:
      | NxtrConf = 'Nexteer Confidential';
      | 
      | sys = bdroot; %handle for the current model ("system")
      | first = get_param(sys,'Created');
      | if(isempty(first))
      |     first = datestr(now,'yyyy');
      | else
      |     first = first(end-3:end);  %year is last four digits
      | end
      | 
      | last = get_param(sys,'LastModifiedDate');
      | if isempty(last)
      |     last = datestr(now,'yyyy');
      | else
      |     last = last(end-3:end);
      | end
      | 
      | if strcmp(first,last)
      |     fprintf('%s -- Copyright %s Nexteer',NxtrConf,first)
      | else
      |     fprintf('%s -- %s%s- %s Nexteer',NxtrConf,char(169),first,last)
      | end
  Ground : Ground
  Terminator : Terminator
  Terminator1 : Terminator
  SigPah_ArgOut : Outport
  wires:
  Ground/1 -> SigPah_ArgOut/1
  LocnKey_ArgIn/1 -> Terminator/1
  SigPah_ArgIn/1 -> Terminator1/1
